simulink model "dlbfuzzy"  (Simulink 8.3)
settings: Solver=ode45  StartTime=0.0  StopTime=10.0  RelTol=1e-3
libraries: fuzblock x2
settings Model: Creator=Administrator  LastModifiedBy=Administrator
settings SolverCC: ZeroCrossControl=DisableAll
settings OptimizationCC: ExpressionDepthLimit=2147483647
settings DebuggingCC: FcnCallInpInsideContextMsg=EnableAllAsWarning

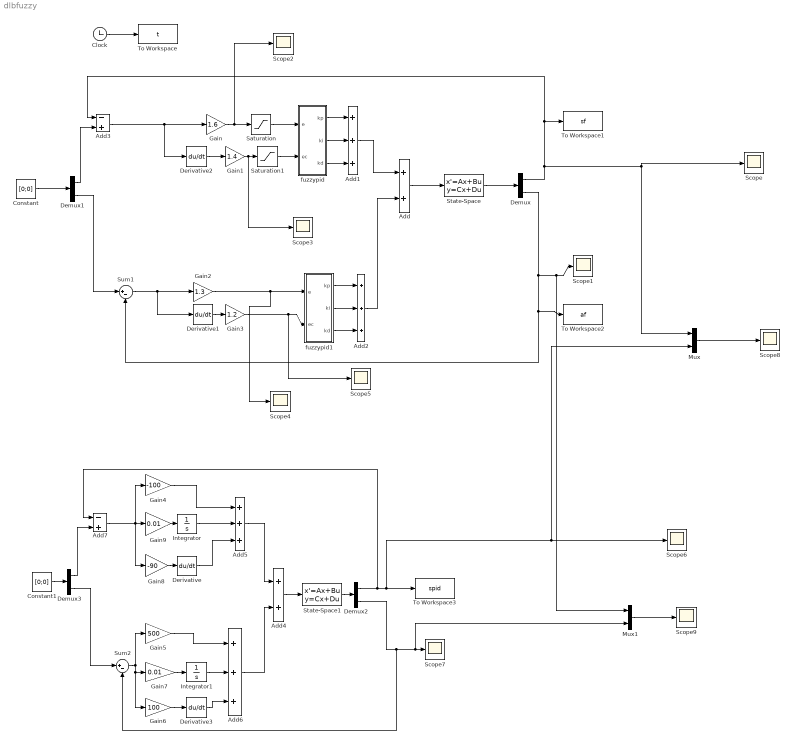
== system dlbfuzzy ==
  Add : Sum
  Add{1..2,5..6} (4 alike) : Sum  Inputs=+++
  Add3 : Sum  Inputs=-+
  Add4 : Sum
  Add7 : Sum  Inputs=-+
  Clock : Clock
  Constant : Constant  Value=[0;0]
  Constant1 : Constant  Value=[0;0]
  Demux{,1..3} (4 alike) : Demux  Outputs=2
  Derivative{,1..3} (4 alike) : Derivative
  Gain : Gain  Gain=1.6
  Gain1 : Gain  Gain=1.4
  Gain2 : Gain  Gain=1.3
  Gain3 : Gain  Gain=1.2
  Gain4 : Gain  Gain=-100
  Gain5 : Gain  Gain=500
  Gain6 : Gain  Gain=100
  Gain7 : Gain  Gain=0.01
  Gain8 : Gain  Gain=-90
  Gain9 : Gain  Gain=0.01
  Integrator : Integrator
  Integrator1 : Integrator
  Mux : Mux  Inputs=2
  Mux1 : Mux  Inputs=2
  Saturation : Saturate  UpperLimit=1  LowerLimit=-1
  Saturation1 : Saturate  UpperLimit=1  LowerLimit=-1
  Scope{,1..9} (10 alike) : Scope
      Scope settings: SaveName=location
      Scope1 settings: SaveName=location1
      Scope2 settings: SaveName=location2
      Scope3 settings: SaveName=location3
      Scope4 settings: SaveName=location4
      Scope5 settings: SaveName=location5
      Scope6 settings: SaveName=location6
      Scope7 settings: SaveName=angle
      Scope8 settings: SaveName=location7
      Scope9 settings: SaveName=location8
  State-Space : StateSpace  A=[0 1 0 0;0 0 0.717 0;0 0 0 1;0 0 15.777 0]  B=[0;0.975;0;1.464]  C=[1 0 0 0;0 0 1 0]  D=[0;0]  X0=[0;0;0.1;0]
  State-Space1 : StateSpace  A=[0 1 0 0;0 0 0.717 0;0 0 0 1;0 0 15.777 0]  B=[0;0.975;0;1.464]  C=[1 0 0 0;0 0 1 0]  D=[0;0]  X0=[0;0;0.1;0]
  Sum1 : Sum  Inputs=|+-
  Sum2 : Sum  Inputs=|+-
  To Workspace : ToWorkspace  VariableName=t  SampleTime=-1
  To Workspace1 : ToWorkspace  VariableName=sf  SampleTime=-1
  To Workspace2 : ToWorkspace  VariableName=af  SampleTime=-1
  To Workspace3 : ToWorkspace  VariableName=spid  SampleTime=-1
  fuzzypid : Subsystem
  fuzzypid1 : Subsystem
  wires:
  Constant/1 -> Demux1/1
  Demux1/1 -> Add3/2
  Add3/1 -> Derivative2/1, Gain/1
  Derivative2/1 -> Gain1/1
  fuzzypid/1(kp) -> Add1/1
  fuzzypid/2(ki) -> Add1/2
  fuzzypid/3(kd) -> Add1/3
  Add1/1 -> Add/1
  Add/1 -> State-Space/1
  State-Space/1 -> Demux/1
  Demux1/2 -> Sum1/1
  Sum1/1 -> Derivative1/1, Gain2/1
  Derivative1/1 -> Gain3/1
  fuzzypid1/1(kp) -> Add2/1
  fuzzypid1/2(ki) -> Add2/2
  fuzzypid1/3(kd) -> Add2/3
  Add2/1 -> Add/2
  Demux/2 -> Mux1/1, Scope1/1, Sum1/2, To Workspace2/1
  Demux/1 -> Scope/1, Mux/1, Add3/1, To Workspace1/1
  Gain/1 -> Scope2/1, Saturation/1
  Gain2/1 -> Scope4/1, fuzzypid1/1(e)
  Gain3/1 -> Scope5/1, fuzzypid1/2(ec)
  Clock/1 -> To Workspace/1
  Saturation/1 -> fuzzypid/1(e)
  Saturation1/1 -> fuzzypid/2(ec)
  Gain1/1 -> Scope3/1, Saturation1/1
  Demux3/2 -> Sum2/1
  Sum2/1 -> Gain6/1, Gain7/1, Gain5/1
  Gain6/1 -> Derivative3/1
  Gain7/1 -> Integrator1/1
  Gain5/1 -> Add6/1
  Demux3/1 -> Add7/2
  Add7/1 -> Gain9/1, Gain4/1, Gain8/1
  Gain8/1 -> Derivative/1
  Gain9/1 -> Integrator/1
  Gain4/1 -> Add5/1
  Add5/1 -> Add4/1
  Add6/1 -> Add4/2
  Add4/1 -> State-Space1/1
  State-Space1/1 -> Demux2/1
  Demux2/2 -> Sum2/2, Mux1/2, Scope7/1
  Constant1/1 -> Demux3/1
  Integrator/1 -> Add5/2
  Derivative/1 -> Add5/3
  Integrator1/1 -> Add6/2
  Derivative3/1 -> Add6/3
  Demux2/1 -> Add7/1, Mux/2, Scope6/1, To Workspace3/1
  Mux/1 -> Scope8/1
  Mux1/1 -> Scope9/1

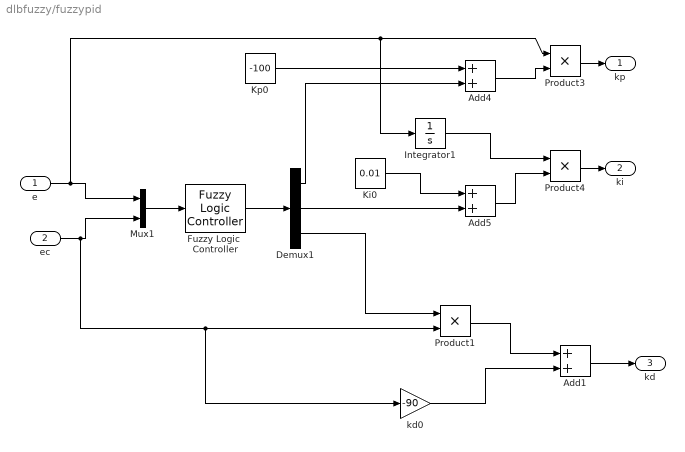
== system dlbfuzzy/fuzzypid ==
  e : Inport
  ec : Inport  Port=2
  Add1 : Sum
  Add4 : Sum
  Add5 : Sum
  Demux1 : Demux  Outputs=3
  Fuzzy Logic  Controller : fuzblock/Fuzzy Logic  Controller  fis=s
  Integrator1 : Integrator
  Ki0 : Constant  Value=0.01
  Kp0 : Constant  Value=-100
  Mux1 : Mux  Inputs=2
  Product1 : Product  RndMeth=Zero
  Product3 : Product  RndMeth=Zero
  Product4 : Product  RndMeth=Zero
  kd0 : Gain  Gain=-90
  kp : Outport
  ki : Outport  Port=2
  kd : Outport  Port=3
  wires:
  Add1/1 -> kd/1
  Product1/1 -> Add1/1
  kd0/1 -> Add1/2
  Demux1/3 -> Product1/1
  Product4/1 -> ki/1
  Product3/1 -> kp/1
  Fuzzy Logic  Controller/1 -> Demux1/1
  Add5/1 -> Product4/2
  Integrator1/1 -> Product4/1
  Ki0/1 -> Add5/1
  Demux1/2 -> Add5/2
  Add4/1 -> Product3/2
  Kp0/1 -> Add4/1
  Demux1/1 -> Add4/2
  Mux1/1 -> Fuzzy Logic  Controller/1
  ec/1 -> kd0/1, Product1/2, Mux1/2
  e/1 -> Integrator1/1, Product3/1, Mux1/1

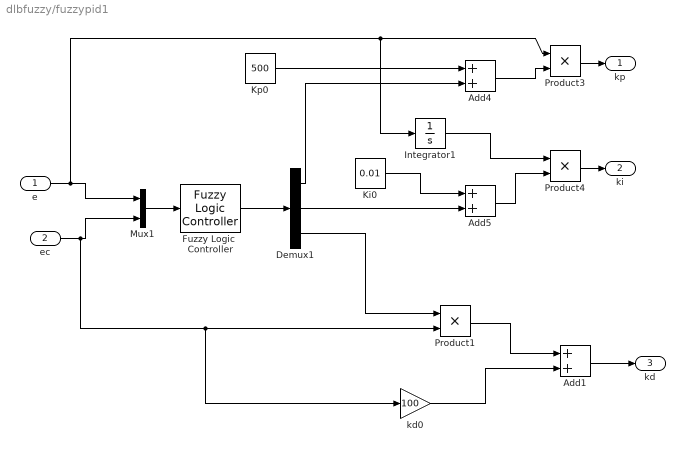
== system dlbfuzzy/fuzzypid1 ==
  e : Inport
  ec : Inport  Port=2
  Add1 : Sum
  Add4 : Sum
  Add5 : Sum
  Demux1 : Demux  Outputs=3
  Fuzzy Logic  Controller : fuzblock/Fuzzy Logic  Controller  fis=angle2
  Integrator1 : Integrator
  Ki0 : Constant  Value=0.01
  Kp0 : Constant  Value=500
  Mux1 : Mux  Inputs=2
  Product1 : Product  RndMeth=Zero
  Product3 : Product  RndMeth=Zero
  Product4 : Product  RndMeth=Zero
  kd0 : Gain  Gain=100
  kp : Outport
  ki : Outport  Port=2
  kd : Outport  Port=3
  wires:
  e/1 -> Mux1/1, Product3/1, Integrator1/1
  ec/1 -> Mux1/2, Product1/2, kd0/1
  Mux1/1 -> Fuzzy Logic  Controller/1
  Demux1/1 -> Add4/2
  Kp0/1 -> Add4/1
  Add4/1 -> Product3/2
  Demux1/2 -> Add5/2
  Ki0/1 -> Add5/1
  Integrator1/1 -> Product4/1
  Add5/1 -> Product4/2
  Fuzzy Logic  Controller/1 -> Demux1/1
  Product3/1 -> kp/1
  Product4/1 -> ki/1
  Demux1/3 -> Product1/1
  kd0/1 -> Add1/2
  Product1/1 -> Add1/1
  Add1/1 -> kd/1
